simulink model "Calibration_IcestorageModel"  (R2018b)
settings: Solver=ode45  StartTime=(-31+16)*24*3600*0  StopTime=(31+29+31+30+31+30+31+31)*24*3600 %23*24*3600  EnableMultiTasking=on
libraries: carnot x43
(part 2 of 2)

== system Calibration_IcestorageModel/Daten Ldf einlesen messdaten1_2011dez_2012aug/InteressanterRest ==
  data : Inport
  Selector : Selector  InputPortWidth=36  IndexOptions=Index vector (dialog)  Indices=[v]  OutputSizes=1
  out : Outport  InitialOutput=0
  wires:
  data/1 -> Selector/1
  Selector/1 -> out/1

== system Calibration_IcestorageModel/Daten Ldf einlesen messdaten1_2011dez_2012aug/InteressanterRest1 ==
  data : Inport
  Selector : Selector  InputPortWidth=36  IndexOptions=Index vector (dialog)  Indices=[v]  OutputSizes=1
  out : Outport  InitialOutput=0
  wires:
  Selector/1 -> out/1
  data/1 -> Selector/1

== system Calibration_IcestorageModel/Daten Ldf einlesen messdaten1_2011dez_2012aug/InteressanterRest2 ==
  data : Inport
  Selector : Selector  InputPortWidth=36  IndexOptions=Index vector (dialog)  Indices=[v]  OutputSizes=1
  out : Outport  InitialOutput=0
  wires:
  data/1 -> Selector/1
  Selector/1 -> out/1

== system Calibration_IcestorageModel/Daten Ldf einlesen messdaten1_2011dez_2012aug/InteressanterRest3 ==
  data : Inport
  Selector : Selector  InputPortWidth=36  IndexOptions=Index vector (dialog)  Indices=[v]  OutputSizes=1
  out : Outport  InitialOutput=0
  wires:
  Selector/1 -> out/1
  data/1 -> Selector/1

== system Calibration_IcestorageModel/Daten Ldf einlesen messdaten1_2011dez_2012aug/Strom ==
  data : Inport
  Selector : Selector  InputPortWidth=36  IndexOptions=Index vector (dialog)  Indices=[v]  OutputSizes=1
  out : Outport  InitialOutput=0
  wires:
  Selector/1 -> out/1
  data/1 -> Selector/1

== system Calibration_IcestorageModel/Daten Ldf einlesen messdaten1_2011dez_2012aug/THO ==
  data : Inport
  Selector : Selector  InputPortWidth=36  IndexOptions=Index vector (dialog)  Indices=[v]  OutputSizes=1
  out : Outport  InitialOutput=0
  wires:
  Selector/1 -> out/1
  data/1 -> Selector/1

== system Calibration_IcestorageModel/Daten Ldf einlesen messdaten1_2011dez_2012aug/converts 4-20mA  to  0-1500W ==
  note: converts
      | 4-20mA  to  0-1500W
  In1 : Inport
  Bias : Bias  Bias=-0.0041
  Gain : Gain  Gain=1/0.0159*1500
  Out1 : Outport
  wires:
  Gain/1 -> Out1/1
  In1/1 -> Bias/1
  Bias/1 -> Gain/1

== system Calibration_IcestorageModel/ice_storage earth-mdl r05/heat exchanger heat pump ==
  Tice : Inport
  Tin : Inport  Port=2
  mdot : Inport  Port=3
  p : Inport  Port=4
  fluid : Inport  Port=5
  mix : Inport  Port=6
  1/(m*cp) : Gain  Gain=1/(1*l_hp*3500)  SaturateOnIntegerOverflow=on  OutDataTypeStr=Inherit: Same as input  ParamDataTypeStr=Inherit: Same as input
  Integrator : Integrator
  Product : Product  Inputs=3  SaturateOnIntegerOverflow=on  InputSameDT=on  OutDataTypeStr=Inherit: Same as first input
  Sum : Sum  Inputs=-+  SaturateOnIntegerOverflow=on  InputSameDT=on  OutDataTypeStr=Inherit: Same as first input
  Sum1 : Sum  Inputs=-+  SaturateOnIntegerOverflow=on  InputSameDT=on  OutDataTypeStr=Inherit: Same as first input
  Sum2 : Sum  Inputs=+-  SaturateOnIntegerOverflow=on  InputSameDT=on  OutDataTypeStr=Inherit: Same as first input
  UA : Gain  Gain="1500/28/9.5*l_hp*25/32            % 1.5 kW at 9 K on a 28 m tube with Da=32 (now Da=25)"  SaturateOnIntegerOverflow=on  OutDataTypeStr=Inherit: Same as input  ParamDataTypeStr=Inherit: Same as input
  heat_capacity : carnot/Basic/Material_Properties/Heat_Capacity  VariantControl=CarlibClassic  INPUTARGUMENTS=state variables (classic)  DEBUGLEVEL=DEBUGLEVEL  MAXTOTALWARNINGS=inf  MAXCONSECUTIVEWARNINGS=inf  WRITETOFILE=0  FILENAME='errors.txt'
      settings: SourceProductName=Carnot
  Qdot2ice : Outport
  Thx_coll : Outport  Port=2
  wires:
  Tin/1 -> Sum/2, heat_capacity/1
  Integrator/1 -> Sum/1, Sum2/1, Thx_coll/1  "Thx_coll"
  Sum1/1 -> 1/(m*cp)/1
  Product/1 -> Sum1/2
  heat_capacity/1 -> Product/3
  Sum/1 -> Product/1
  Sum2/1 -> UA/1
  mdot/1 -> Product/2
  p/1 -> heat_capacity/2
  fluid/1 -> heat_capacity/3
  mix/1 -> heat_capacity/4
  Tice/1 -> Sum2/2
  1/(m*cp)/1 -> Integrator/1
  UA/1 -> Sum1/1, Qdot2ice/1

== system Calibration_IcestorageModel/ice_storage earth-mdl r05/heat exchanger solar ==
  Tice : Inport
  Tin : Inport  Port=2
  mdot : Inport  Port=3
  p : Inport  Port=4
  fluid : Inport  Port=5
  mix : Inport  Port=6
  1/(m*cp) : Gain  Gain=1/(1*l_solar*3500)  SaturateOnIntegerOverflow=on  OutDataTypeStr=Inherit: Same as input  ParamDataTypeStr=Inherit: Same as input
  Integrator : Integrator
  Product : Product  Inputs=3  SaturateOnIntegerOverflow=on  InputSameDT=on  OutDataTypeStr=Inherit: Same as first input
  Sum : Sum  Inputs=-+  SaturateOnIntegerOverflow=on  InputSameDT=on  OutDataTypeStr=Inherit: Same as first input
  Sum1 : Sum  Inputs=-+  SaturateOnIntegerOverflow=on  InputSameDT=on  OutDataTypeStr=Inherit: Same as first input
  Sum2 : Sum  Inputs=+-  SaturateOnIntegerOverflow=on  InputSameDT=on  OutDataTypeStr=Inherit: Same as first input
  UA : Gain  Gain="1500/28/9.5*l_solar*25/32            % 1.5 kW at 9 K on a 28 m tube with Da=32 (now Da=25)"  SaturateOnIntegerOverflow=on  OutDataTypeStr=Inherit: Same as input  ParamDataTypeStr=Inherit: Same as input
  heat_capacity : carnot/Basic/Material_Properties/Heat_Capacity  VariantControl=CarlibClassic  INPUTARGUMENTS=state variables (classic)  DEBUGLEVEL=DEBUGLEVEL  MAXTOTALWARNINGS=inf  MAXCONSECUTIVEWARNINGS=inf  WRITETOFILE=0  FILENAME='errors.txt'
      settings: SourceProductName=Carnot
  Qdot2ice : Outport
  Thx_coll : Outport  Port=2
  wires:
  Tice/1 -> Sum2/2
  mix/1 -> heat_capacity/4
  fluid/1 -> heat_capacity/3
  p/1 -> heat_capacity/2
  mdot/1 -> Product/2
  Sum2/1 -> UA/1
  Sum/1 -> Product/1
  heat_capacity/1 -> Product/3
  Product/1 -> Sum1/2
  Sum1/1 -> 1/(m*cp)/1
  Integrator/1 -> Thx_coll/1, Sum2/1, Sum/1  "Thx_coll"
  Tin/1 -> heat_capacity/1, Sum/2
  1/(m*cp)/1 -> Integrator/1
  UA/1 -> Qdot2ice/1, Sum1/1

== system Calibration_IcestorageModel/ice_storage earth-mdl r05/undisturbed ground temperature1 ==
  Fcn : Fcn  Expr=u(1) - u(2)*exp(-u(3)/u(4))*cos(2*pi*(u(5)-u(6)*3600)/(365*24*3600) - u(3)/u(4)) + 0.03*u(3)
  Mux : Mux  Inputs=6
  Tmeanoutside : Constant  Value=Tmeanoutside
  delta_grd : Constant  Value=delta_grd
  deltathetae : Constant  Value=deltathetae
  depth of center of wall : Constant  Value=ztilde
  time : Clock
  tshift : Constant  Value=tshift
  Tearth : Outport
  wires:
  Fcn/1 -> Tearth/1
  Mux/1 -> Fcn/1
  tshift/1 -> Mux/6
  time/1 -> Mux/5
  delta_grd/1 -> Mux/4
  depth of center of wall/1 -> Mux/3
  deltathetae/1 -> Mux/2
  Tmeanoutside/1 -> Mux/1

== system Calibration_IcestorageModel/ice_storage new earth+HX-mdl_r06/heat exchanger solar ==
  Tice : Inport
  Tin : Inport  Port=2
  mdot : Inport  Port=3
  p : Inport  Port=4
  fluid : Inport  Port=5
  mix : Inport  Port=6
  1/(m*cp) : Gain  Gain=1/(1*l_solar*3500)  SaturateOnIntegerOverflow=on  OutDataTypeStr=Inherit: Same as input  ParamDataTypeStr=Inherit: Same as input
  Integrator : Integrator
  Product : Product  Inputs=3  SaturateOnIntegerOverflow=on  InputSameDT=on  OutDataTypeStr=Inherit: Same as first input
  Sum : Sum  Inputs=-+  SaturateOnIntegerOverflow=on  InputSameDT=on  OutDataTypeStr=Inherit: Same as first input
  Sum1 : Sum  Inputs=-+  SaturateOnIntegerOverflow=on  InputSameDT=on  OutDataTypeStr=Inherit: Same as first input
  Sum2 : Sum  Inputs=+-  SaturateOnIntegerOverflow=on  InputSameDT=on  OutDataTypeStr=Inherit: Same as first input
  UA : Gain  Gain="1500/28/9.5*l_solar*25/32            % 1.5 kW at 9 K on a 28 m tube with Da=32 (now Da=25)"  SaturateOnIntegerOverflow=on  OutDataTypeStr=Inherit: Same as input  ParamDataTypeStr=Inherit: Same as input
  heat_capacity : carnot/Basic/Material_Properties/Heat_Capacity  VariantControl=CarlibClassic  INPUTARGUMENTS=state variables (classic)  DEBUGLEVEL=DEBUGLEVEL  MAXTOTALWARNINGS=inf  MAXCONSECUTIVEWARNINGS=inf  WRITETOFILE=0  FILENAME='errors.txt'
      settings: SourceProductName=Carnot
  Qdot2ice : Outport
  Thx_coll : Outport  Port=2
  wires:
  Tin/1 -> Sum/2, heat_capacity/1
  Integrator/1 -> Sum/1, Sum2/1, Thx_coll/1  "Thx_coll"
  1/(m*cp)/1 -> Integrator/1
  Sum1/1 -> 1/(m*cp)/1
  Product/1 -> Sum1/2
  heat_capacity/1 -> Product/3
  Sum/1 -> Product/1
  Sum2/1 -> UA/1
  UA/1 -> Qdot2ice/1, Sum1/1
  mdot/1 -> Product/2
  p/1 -> heat_capacity/2
  fluid/1 -> heat_capacity/3
  mix/1 -> heat_capacity/4
  Tice/1 -> Sum2/2

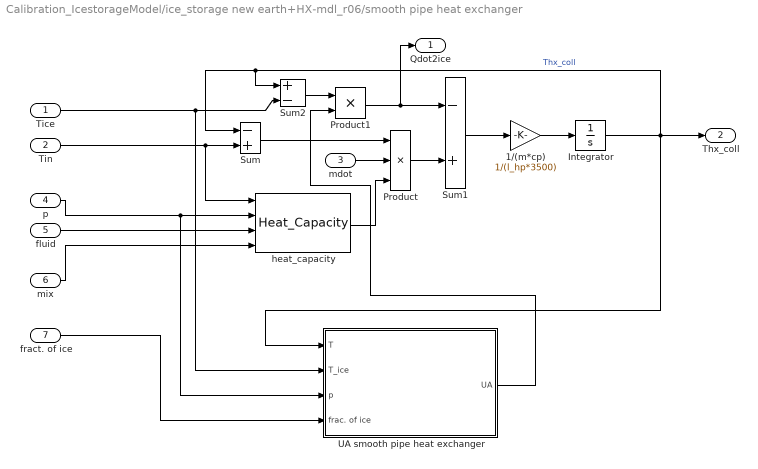
== system Calibration_IcestorageModel/ice_storage new earth+HX-mdl_r06/smooth pipe heat exchanger ==
  Tice : Inport
  Tin : Inport  Port=2
  mdot : Inport  Port=3
  p : Inport  Port=4
  fluid : Inport  Port=5
  mix : Inport  Port=6
  fract. of ice : Inport  Port=7
  1/(m*cp) : Gain  Gain=1/(l_hp*3500)  SaturateOnIntegerOverflow=on  OutDataTypeStr=Inherit: Same as input  ParamDataTypeStr=Inherit: Same as input
  Integrator : Integrator
  Product : Product  Inputs=3  SaturateOnIntegerOverflow=on  InputSameDT=on  OutDataTypeStr=Inherit: Same as first input
  Product1 : Product  RndMeth=Zero
  Sum : Sum  Inputs=-+  SaturateOnIntegerOverflow=on  InputSameDT=on  OutDataTypeStr=Inherit: Same as first input
  Sum1 : Sum  Inputs=-+  SaturateOnIntegerOverflow=on  InputSameDT=on  OutDataTypeStr=Inherit: Same as first input
  Sum2 : Sum  Inputs=+-  SaturateOnIntegerOverflow=on  InputSameDT=on  OutDataTypeStr=Inherit: Same as first input
  UA smooth pipe heat exchanger : Subsystem
      mask help:
      | Calculates the  heat exchange of a smooth pipe heat exchanger.
      | Calls calls the function "grashof" in the CARNOT library "carlib".
      | Definition of the fluid types
      | fluid-ID  material           remarks on fluid mix
      | 1           water              vapourcontent in the 2-phase region
      | 2           air                   is (kg water) / (kg air)
      | 3           cotton oil
      | 4           silicone oil
      | 5           water-glycol    gives the volume partition [0..1] of glycol
  heat_capacity : carnot/Basic/Material_Properties/Heat_Capacity  VariantControl=CarlibClassic  INPUTARGUMENTS=state variables (classic)  DEBUGLEVEL=DEBUGLEVEL  MAXTOTALWARNINGS=inf  MAXCONSECUTIVEWARNINGS=inf  WRITETOFILE=0  FILENAME='errors.txt'
      settings: SourceProductName=Carnot
  Qdot2ice : Outport
  Thx_coll : Outport  Port=2
  wires:
  fract. of ice/1 -> UA smooth pipe heat exchanger/4(frac. of ice)
  Product1/1 -> Sum1/1, Qdot2ice/1
  UA smooth pipe heat exchanger/1(UA) -> Product1/2
  Tin/1 -> Sum/2, heat_capacity/1
  Integrator/1 -> Sum/1, Sum2/1, Thx_coll/1, UA smooth pipe heat exchanger/1(T)  "Thx_coll"
  Sum1/1 -> 1/(m*cp)/1
  Product/1 -> Sum1/2
  heat_capacity/1 -> Product/3
  Sum/1 -> Product/1
  Sum2/1 -> Product1/1
  mdot/1 -> Product/2
  p/1 -> UA smooth pipe heat exchanger/3(p), heat_capacity/2
  fluid/1 -> heat_capacity/3
  mix/1 -> heat_capacity/4
  Tice/1 -> UA smooth pipe heat exchanger/2(T_ice), Sum2/2
  1/(m*cp)/1 -> Integrator/1

== system Calibration_IcestorageModel/ice_storage new earth+HX-mdl_r06/undisturbed ground temperature ==
  Fcn : Fcn  Expr=u(1) - u(2)*exp(-u(3)/u(4))*cos(2*pi*(u(5)-u(6)*3600)/(365*24*3600) - u(3)/u(4)) + 0.03*u(3)
  Mux : Mux  Inputs=6
  Tmeanoutside : Constant  Value=Tmeanoutside
  delta_grd : Constant  Value=delta_grd
  deltathetae : Constant  Value=deltathetae
  depth of center of wall : Constant  Value=ztilde
  time : Clock
  tshift : Constant  Value=tshift
  Tearth : Outport
  wires:
  Fcn/1 -> Tearth/1
  Mux/1 -> Fcn/1
  tshift/1 -> Mux/6
  time/1 -> Mux/5
  delta_grd/1 -> Mux/4
  depth of center of wall/1 -> Mux/3
  deltathetae/1 -> Mux/2
  Tmeanoutside/1 -> Mux/1

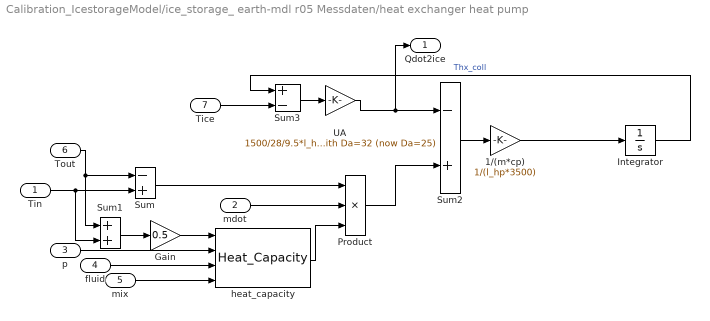
== system Calibration_IcestorageModel/ice_storage_ earth-mdl r05 Messdaten/heat exchanger heat pump ==
  Tin : Inport
  mdot : Inport  Port=2
  p : Inport  Port=3
  fluid : Inport  Port=4
  mix : Inport  Port=5
  Tout : Inport  Port=6
  Tice : Inport  Port=7
  1/(m*cp) : Gain  Gain=1/(l_hp*3500)  SaturateOnIntegerOverflow=on  OutDataTypeStr=Inherit: Same as input  ParamDataTypeStr=Inherit: Same as input
  Gain : Gain  Gain=0.5
  Integrator : Integrator
  Product : Product  Inputs=3  SaturateOnIntegerOverflow=on  InputSameDT=on  OutDataTypeStr=Inherit: Same as first input
  Sum : Sum  Inputs=-+  SaturateOnIntegerOverflow=on  InputSameDT=on  OutDataTypeStr=Inherit: Same as first input
  Sum1 : Sum  SaturateOnIntegerOverflow=on  InputSameDT=on  OutDataTypeStr=Inherit: Same as first input
  Sum2 : Sum  Inputs=-+  SaturateOnIntegerOverflow=on  InputSameDT=on  OutDataTypeStr=Inherit: Same as first input
  Sum3 : Sum  Inputs=+-  SaturateOnIntegerOverflow=on  InputSameDT=on  OutDataTypeStr=Inherit: Same as first input
  UA : Gain  Gain="1500/28/9.5*l_hp*25/32            % 1.5 kW at 9 K on a 28 m tube with Da=32 (now Da=25)"  SaturateOnIntegerOverflow=on  OutDataTypeStr=Inherit: Same as input  ParamDataTypeStr=Inherit: Same as input
  heat_capacity : carnot/Basic/Material_Properties/Heat_Capacity  VariantControl=CarlibClassic  INPUTARGUMENTS=state variables (classic)  DEBUGLEVEL=DEBUGLEVEL  MAXTOTALWARNINGS=inf  MAXCONSECUTIVEWARNINGS=inf  WRITETOFILE=0  FILENAME='errors.txt'
      settings: SourceProductName=Carnot
  Qdot2ice : Outport
  wires:
  Gain/1 -> heat_capacity/1
  Sum1/1 -> Gain/1
  Tout/1 -> Sum1/1, Sum/1
  Tin/1 -> Sum1/2, Sum/2
  heat_capacity/1 -> Product/3
  Sum/1 -> Product/1
  mdot/1 -> Product/2
  p/1 -> heat_capacity/2
  fluid/1 -> heat_capacity/3
  mix/1 -> heat_capacity/4
  UA/1 -> Sum2/1, Qdot2ice/1
  Integrator/1 -> Sum3/1  "Thx_coll"
  Sum2/1 -> 1/(m*cp)/1
  Sum3/1 -> UA/1
  1/(m*cp)/1 -> Integrator/1
  Product/1 -> Sum2/2
  Tice/1 -> Sum3/2

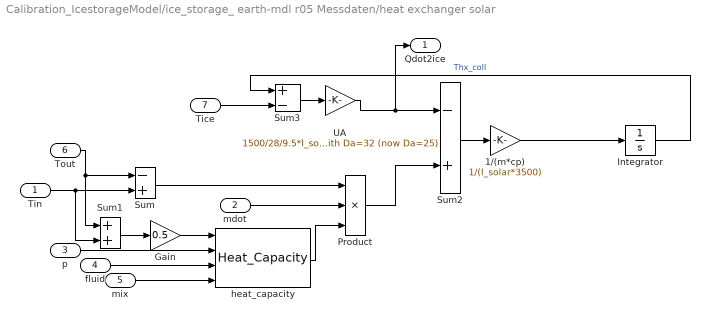
== system Calibration_IcestorageModel/ice_storage_ earth-mdl r05 Messdaten/heat exchanger solar ==
  Tin : Inport
  mdot : Inport  Port=2
  p : Inport  Port=3
  fluid : Inport  Port=4
  mix : Inport  Port=5
  Tout : Inport  Port=6
  Tice : Inport  Port=7
  1/(m*cp) : Gain  Gain=1/(l_solar*3500)  SaturateOnIntegerOverflow=on  OutDataTypeStr=Inherit: Same as input  ParamDataTypeStr=Inherit: Same as input
  Gain : Gain  Gain=0.5
  Integrator : Integrator
  Product : Product  Inputs=3  SaturateOnIntegerOverflow=on  InputSameDT=on  OutDataTypeStr=Inherit: Same as first input
  Sum : Sum  Inputs=-+  SaturateOnIntegerOverflow=on  InputSameDT=on  OutDataTypeStr=Inherit: Same as first input
  Sum1 : Sum  SaturateOnIntegerOverflow=on  InputSameDT=on  OutDataTypeStr=Inherit: Same as first input
  Sum2 : Sum  Inputs=-+  SaturateOnIntegerOverflow=on  InputSameDT=on  OutDataTypeStr=Inherit: Same as first input
  Sum3 : Sum  Inputs=+-  SaturateOnIntegerOverflow=on  InputSameDT=on  OutDataTypeStr=Inherit: Same as first input
  UA : Gain  Gain="1500/28/9.5*l_solar*25/32            % 1.5 kW at 9 K on a 28 m tube with Da=32 (now Da=25)"  SaturateOnIntegerOverflow=on  OutDataTypeStr=Inherit: Same as input  ParamDataTypeStr=Inherit: Same as input
  heat_capacity : carnot/Basic/Material_Properties/Heat_Capacity  VariantControl=CarlibClassic  INPUTARGUMENTS=state variables (classic)  DEBUGLEVEL=DEBUGLEVEL  MAXTOTALWARNINGS=inf  MAXCONSECUTIVEWARNINGS=inf  WRITETOFILE=0  FILENAME='errors.txt'
      settings: SourceProductName=Carnot
  Qdot2ice : Outport
  wires:
  Tice/1 -> Sum3/2
  Product/1 -> Sum2/2
  1/(m*cp)/1 -> Integrator/1
  Sum3/1 -> UA/1
  Sum2/1 -> 1/(m*cp)/1
  Integrator/1 -> Sum3/1  "Thx_coll"
  UA/1 -> Qdot2ice/1, Sum2/1
  mix/1 -> heat_capacity/4
  fluid/1 -> heat_capacity/3
  p/1 -> heat_capacity/2
  mdot/1 -> Product/2
  Sum/1 -> Product/1
  heat_capacity/1 -> Product/3
  Tin/1 -> Sum/2, Sum1/2
  Tout/1 -> Sum/1, Sum1/1
  Sum1/1 -> Gain/1
  Gain/1 -> heat_capacity/1

== system Calibration_IcestorageModel/ice_storage_ earth-mdl r05 Messdaten/undisturbed ground temperature1 ==
  Fcn : Fcn  Expr=u(1) - u(2)*exp(-u(3)/u(4))*cos(2*pi*(u(5)-u(6)*3600)/(365*24*3600) - u(3)/u(4)) + 0.03*u(3)
  Mux : Mux  Inputs=6
  Tmeanoutside : Constant  Value=Tmeanoutside
  delta_grd : Constant  Value=delta_grd
  deltathetae : Constant  Value=deltathetae
  depth of center of wall : Constant  Value=ztilde
  time : Clock
  tshift : Constant  Value=tshift
  Tearth : Outport
  wires:
  Fcn/1 -> Tearth/1
  Mux/1 -> Fcn/1
  tshift/1 -> Mux/6
  time/1 -> Mux/5
  delta_grd/1 -> Mux/4
  depth of center of wall/1 -> Mux/3
  deltathetae/1 -> Mux/2
  Tmeanoutside/1 -> Mux/1

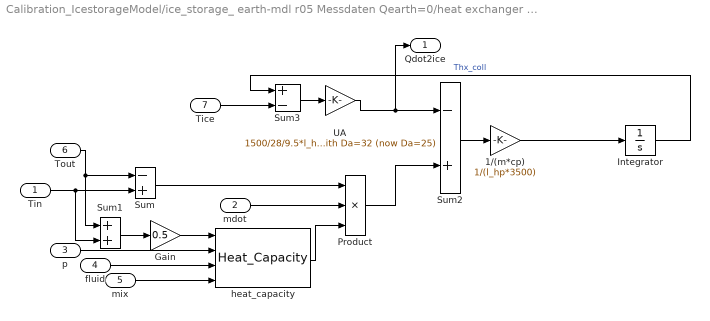
== system Calibration_IcestorageModel/ice_storage_ earth-mdl r05 Messdaten Qearth=0/heat exchanger heat pump ==
  Tin : Inport
  mdot : Inport  Port=2
  p : Inport  Port=3
  fluid : Inport  Port=4
  mix : Inport  Port=5
  Tout : Inport  Port=6
  Tice : Inport  Port=7
  1/(m*cp) : Gain  Gain=1/(l_hp*3500)  SaturateOnIntegerOverflow=on  OutDataTypeStr=Inherit: Same as input  ParamDataTypeStr=Inherit: Same as input
  Gain : Gain  Gain=0.5
  Integrator : Integrator
  Product : Product  Inputs=3  SaturateOnIntegerOverflow=on  InputSameDT=on  OutDataTypeStr=Inherit: Same as first input
  Sum : Sum  Inputs=-+  SaturateOnIntegerOverflow=on  InputSameDT=on  OutDataTypeStr=Inherit: Same as first input
  Sum1 : Sum  SaturateOnIntegerOverflow=on  InputSameDT=on  OutDataTypeStr=Inherit: Same as first input
  Sum2 : Sum  Inputs=-+  SaturateOnIntegerOverflow=on  InputSameDT=on  OutDataTypeStr=Inherit: Same as first input
  Sum3 : Sum  Inputs=+-  SaturateOnIntegerOverflow=on  InputSameDT=on  OutDataTypeStr=Inherit: Same as first input
  UA : Gain  Gain="1500/28/9.5*l_hp*25/32            % 1.5 kW at 9 K on a 28 m tube with Da=32 (now Da=25)"  SaturateOnIntegerOverflow=on  OutDataTypeStr=Inherit: Same as input  ParamDataTypeStr=Inherit: Same as input
  heat_capacity : carnot/Basic/Material_Properties/Heat_Capacity  VariantControl=CarlibClassic  INPUTARGUMENTS=state variables (classic)  DEBUGLEVEL=DEBUGLEVEL  MAXTOTALWARNINGS=inf  MAXCONSECUTIVEWARNINGS=inf  WRITETOFILE=0  FILENAME='errors.txt'
      settings: SourceProductName=Carnot
  Qdot2ice : Outport
  wires:
  Tice/1 -> Sum3/2
  Product/1 -> Sum2/2
  1/(m*cp)/1 -> Integrator/1
  Sum3/1 -> UA/1
  Sum2/1 -> 1/(m*cp)/1
  Integrator/1 -> Sum3/1  "Thx_coll"
  UA/1 -> Qdot2ice/1, Sum2/1
  mix/1 -> heat_capacity/4
  fluid/1 -> heat_capacity/3
  p/1 -> heat_capacity/2
  mdot/1 -> Product/2
  Sum/1 -> Product/1
  heat_capacity/1 -> Product/3
  Tin/1 -> Sum/2, Sum1/2
  Tout/1 -> Sum/1, Sum1/1
  Sum1/1 -> Gain/1
  Gain/1 -> heat_capacity/1

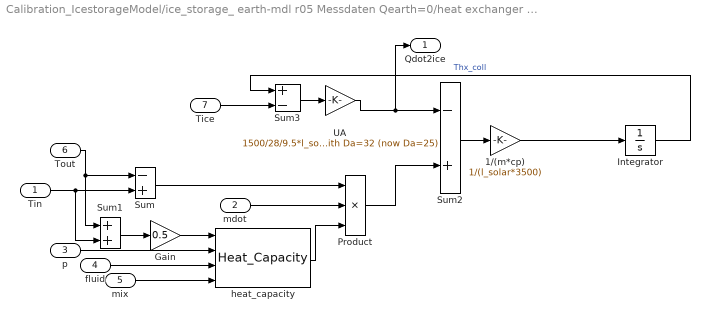
== system Calibration_IcestorageModel/ice_storage_ earth-mdl r05 Messdaten Qearth=0/heat exchanger solar ==
  Tin : Inport
  mdot : Inport  Port=2
  p : Inport  Port=3
  fluid : Inport  Port=4
  mix : Inport  Port=5
  Tout : Inport  Port=6
  Tice : Inport  Port=7
  1/(m*cp) : Gain  Gain=1/(l_solar*3500)  SaturateOnIntegerOverflow=on  OutDataTypeStr=Inherit: Same as input  ParamDataTypeStr=Inherit: Same as input
  Gain : Gain  Gain=0.5
  Integrator : Integrator
  Product : Product  Inputs=3  SaturateOnIntegerOverflow=on  InputSameDT=on  OutDataTypeStr=Inherit: Same as first input
  Sum : Sum  Inputs=-+  SaturateOnIntegerOverflow=on  InputSameDT=on  OutDataTypeStr=Inherit: Same as first input
  Sum1 : Sum  SaturateOnIntegerOverflow=on  InputSameDT=on  OutDataTypeStr=Inherit: Same as first input
  Sum2 : Sum  Inputs=-+  SaturateOnIntegerOverflow=on  InputSameDT=on  OutDataTypeStr=Inherit: Same as first input
  Sum3 : Sum  Inputs=+-  SaturateOnIntegerOverflow=on  InputSameDT=on  OutDataTypeStr=Inherit: Same as first input
  UA : Gain  Gain="1500/28/9.5*l_solar*25/32            % 1.5 kW at 9 K on a 28 m tube with Da=32 (now Da=25)"  SaturateOnIntegerOverflow=on  OutDataTypeStr=Inherit: Same as input  ParamDataTypeStr=Inherit: Same as input
  heat_capacity : carnot/Basic/Material_Properties/Heat_Capacity  VariantControl=CarlibClassic  INPUTARGUMENTS=state variables (classic)  DEBUGLEVEL=DEBUGLEVEL  MAXTOTALWARNINGS=inf  MAXCONSECUTIVEWARNINGS=inf  WRITETOFILE=0  FILENAME='errors.txt'
      settings: SourceProductName=Carnot
  Qdot2ice : Outport
  wires:
  Gain/1 -> heat_capacity/1
  Sum1/1 -> Gain/1
  Tout/1 -> Sum1/1, Sum/1
  Tin/1 -> Sum1/2, Sum/2
  heat_capacity/1 -> Product/3
  Sum/1 -> Product/1
  mdot/1 -> Product/2
  p/1 -> heat_capacity/2
  fluid/1 -> heat_capacity/3
  mix/1 -> heat_capacity/4
  UA/1 -> Sum2/1, Qdot2ice/1
  Integrator/1 -> Sum3/1  "Thx_coll"
  Sum2/1 -> 1/(m*cp)/1
  Sum3/1 -> UA/1
  1/(m*cp)/1 -> Integrator/1
  Product/1 -> Sum2/2
  Tice/1 -> Sum3/2

== system Calibration_IcestorageModel/ice_storage_ earth-mdl r05 Messdaten Qearth=0/undisturbed ground temperature1 ==
  Fcn : Fcn  Expr=u(1) - u(2)*exp(-u(3)/u(4))*cos(2*pi*(u(5)-u(6)*3600)/(365*24*3600) - u(3)/u(4)) + 0.03*u(3)
  Mux : Mux  Inputs=6
  Tmeanoutside : Constant  Value=Tmeanoutside
  delta_grd : Constant  Value=delta_grd
  deltathetae : Constant  Value=deltathetae
  depth of center of wall : Constant  Value=ztilde
  time : Clock
  tshift : Constant  Value=tshift
  Tearth : Outport
  wires:
  Tmeanoutside/1 -> Mux/1
  deltathetae/1 -> Mux/2
  depth of center of wall/1 -> Mux/3
  delta_grd/1 -> Mux/4
  time/1 -> Mux/5
  tshift/1 -> Mux/6
  Mux/1 -> Fcn/1
  Fcn/1 -> Tearth/1

== system Calibration_IcestorageModel/ice_storage_r04 Messdaten/heat exchanger heat pump ==
  Tin : Inport
  mdot : Inport  Port=2
  p : Inport  Port=3
  fluid : Inport  Port=4
  mix : Inport  Port=5
  Tout : Inport  Port=6
  Tice : Inport  Port=7
  1/(m*cp) : Gain  Gain=1/(l_hp*3500)  SaturateOnIntegerOverflow=on  OutDataTypeStr=Inherit: Same as input  ParamDataTypeStr=Inherit: Same as input
  Gain : Gain  Gain=0.5
  Integrator : Integrator
  Product : Product  Inputs=3  SaturateOnIntegerOverflow=on  InputSameDT=on  OutDataTypeStr=Inherit: Same as first input
  Sum : Sum  Inputs=-+  SaturateOnIntegerOverflow=on  InputSameDT=on  OutDataTypeStr=Inherit: Same as first input
  Sum1 : Sum  SaturateOnIntegerOverflow=on  InputSameDT=on  OutDataTypeStr=Inherit: Same as first input
  Sum2 : Sum  Inputs=-+  SaturateOnIntegerOverflow=on  InputSameDT=on  OutDataTypeStr=Inherit: Same as first input
  Sum3 : Sum  Inputs=+-  SaturateOnIntegerOverflow=on  InputSameDT=on  OutDataTypeStr=Inherit: Same as first input
  UA : Gain  Gain="1500/28/9.5*l_hp*25/32            % 1.5 kW at 9 K on a 28 m tube with Da=32 (now Da=25)"  SaturateOnIntegerOverflow=on  OutDataTypeStr=Inherit: Same as input  ParamDataTypeStr=Inherit: Same as input
  heat_capacity : carnot/Basic/Material_Properties/Heat_Capacity  VariantControl=CarlibClassic  INPUTARGUMENTS=state variables (classic)  DEBUGLEVEL=DEBUGLEVEL  MAXTOTALWARNINGS=inf  MAXCONSECUTIVEWARNINGS=inf  WRITETOFILE=0  FILENAME='errors.txt'
      settings: SourceProductName=Carnot
  Qdot2ice : Outport
  wires:
  Gain/1 -> heat_capacity/1
  Sum1/1 -> Gain/1
  Tout/1 -> Sum1/1, Sum/1
  Tin/1 -> Sum1/2, Sum/2
  heat_capacity/1 -> Product/3
  Sum/1 -> Product/1
  mdot/1 -> Product/2
  p/1 -> heat_capacity/2
  fluid/1 -> heat_capacity/3
  mix/1 -> heat_capacity/4
  UA/1 -> Sum2/1, Qdot2ice/1
  Integrator/1 -> Sum3/1  "Thx_coll"
  Sum2/1 -> 1/(m*cp)/1
  Sum3/1 -> UA/1
  1/(m*cp)/1 -> Integrator/1
  Product/1 -> Sum2/2
  Tice/1 -> Sum3/2

== system Calibration_IcestorageModel/ice_storage_r04 Messdaten/heat exchanger solar ==
  Tin : Inport
  mdot : Inport  Port=2
  p : Inport  Port=3
  fluid : Inport  Port=4
  mix : Inport  Port=5
  Tout : Inport  Port=6
  Tice : Inport  Port=7
  1/(m*cp) : Gain  Gain=1/(l_solar*3500)  SaturateOnIntegerOverflow=on  OutDataTypeStr=Inherit: Same as input  ParamDataTypeStr=Inherit: Same as input
  Gain : Gain  Gain=0.5
  Integrator : Integrator
  Product : Product  Inputs=3  SaturateOnIntegerOverflow=on  InputSameDT=on  OutDataTypeStr=Inherit: Same as first input
  Sum : Sum  Inputs=-+  SaturateOnIntegerOverflow=on  InputSameDT=on  OutDataTypeStr=Inherit: Same as first input
  Sum1 : Sum  SaturateOnIntegerOverflow=on  InputSameDT=on  OutDataTypeStr=Inherit: Same as first input
  Sum2 : Sum  Inputs=-+  SaturateOnIntegerOverflow=on  InputSameDT=on  OutDataTypeStr=Inherit: Same as first input
  Sum3 : Sum  Inputs=+-  SaturateOnIntegerOverflow=on  InputSameDT=on  OutDataTypeStr=Inherit: Same as first input
  UA : Gain  Gain="1500/28/9.5*l_solar*25/32            % 1.5 kW at 9 K on a 28 m tube with Da=32 (now Da=25)"  SaturateOnIntegerOverflow=on  OutDataTypeStr=Inherit: Same as input  ParamDataTypeStr=Inherit: Same as input
  heat_capacity : carnot/Basic/Material_Properties/Heat_Capacity  VariantControl=CarlibClassic  INPUTARGUMENTS=state variables (classic)  DEBUGLEVEL=DEBUGLEVEL  MAXTOTALWARNINGS=inf  MAXCONSECUTIVEWARNINGS=inf  WRITETOFILE=0  FILENAME='errors.txt'
      settings: SourceProductName=Carnot
  Qdot2ice : Outport
  wires:
  Tice/1 -> Sum3/2
  Product/1 -> Sum2/2
  1/(m*cp)/1 -> Integrator/1
  Sum3/1 -> UA/1
  Sum2/1 -> 1/(m*cp)/1
  Integrator/1 -> Sum3/1  "Thx_coll"
  UA/1 -> Qdot2ice/1, Sum2/1
  mix/1 -> heat_capacity/4
  fluid/1 -> heat_capacity/3
  p/1 -> heat_capacity/2
  mdot/1 -> Product/2
  Sum/1 -> Product/1
  heat_capacity/1 -> Product/3
  Tin/1 -> Sum/2, Sum1/2
  Tout/1 -> Sum/1, Sum1/1
  Sum1/1 -> Gain/1
  Gain/1 -> heat_capacity/1

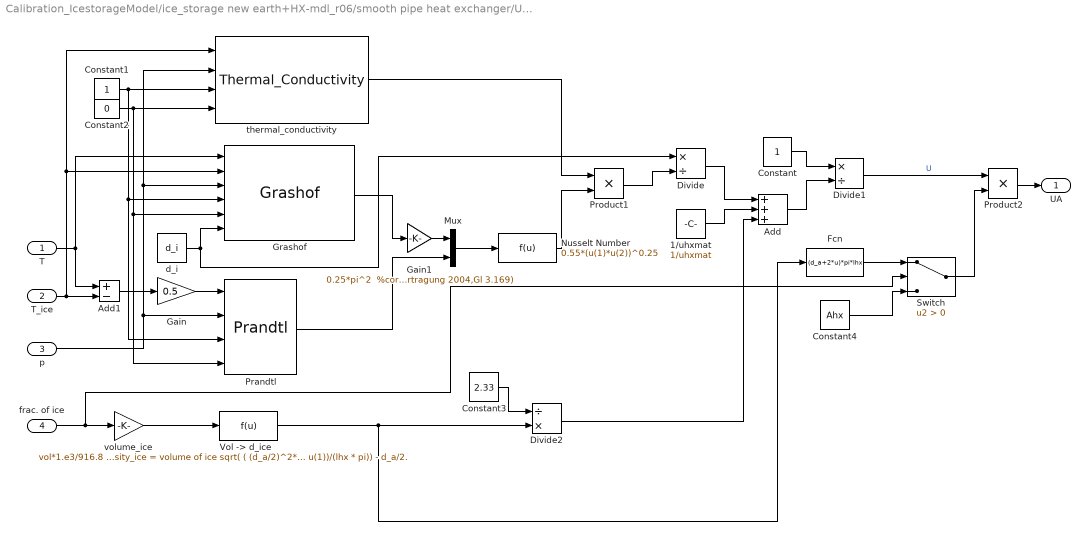
== system Calibration_IcestorageModel/ice_storage new earth+HX-mdl_r06/smooth pipe heat exchanger/UA smooth pipe heat exchanger ==
  T : Inport
  T_ice : Inport  Port=2
  p : Inport  Port=3
  frac. of ice : Inport  Port=4
  1/uhxmat : Constant  Value=1/uhxmat
  Add : Sum  Inputs=+++
  Add1 : Sum  Inputs=+-
  Constant : Constant
  Constant1 : Constant
  Constant2 : Constant  Value=0
  Constant3 : Constant  Value=2.33
  Constant4 : Constant  Value=Ahx
  Divide : Product  Inputs=*/
  Divide1 : Product  Inputs=*/
  Divide2 : Product  Inputs=/*
  Fcn : Fcn  Expr=(d_a+2*u)*pi*lhx
  Gain : Gain  Gain=0.5
  Gain1 : Gain  Gain="0.25*pi^2  %correction for horizontal pipe (Wagner Wärmeübertragung 2004,Gl 3.169)"
  Grashof : carnot/Basic/Hydraulics/Grashof  VariantControl=CarlibClassic  DEBUGLEVEL=WARNINGLEVEL  MAXTOTALMESSAGES=inf  MAXCONSECUTIVEMESSAGES=inf  WRITETOFILE=0  FILENAME='errors.txt'
      settings: SourceProductName=Carnot
  Mux : Mux  Inputs=2
  Nusselt Number : Fcn  Expr=0.55*(u(1)*u(2))^0.25
  Prandtl : carnot/Basic/Hydraulics/Prandtl  VariantControl=CarlibClassic  INPUTARGUMENTS=state variables (classic)  DEBUGLEVEL=WARNINGLEVEL  MAXTOTALMESSAGES=inf  MAXCONSECUTIVEMESSAGES=inf  WRITETOFILE=0  FILENAME='errors.txt'
      settings: SourceProductName=Carnot
  Product1 : Product  RndMeth=Zero
  Product2 : Product  RndMeth=Zero
  Switch : Switch  Criteria=u2 > Threshold
  "Vol -> d_ice" : Fcn  Expr=sqrt( ( (d_a/2)^2*pi*lhx + u(1))/(lhx * pi)) - d_a/2.
  d_i : Constant  Value=d_i
  thermal_conductivity : carnot/Basic/Material_Properties/Thermal_Conductivity  VariantControl=CarlibClassic  INPUTARGUMENTS=state variables (classic)  DEBUGLEVEL=WARNINGLEVEL  MAXTOTALMESSAGES=inf  MAXCONSECUTIVEMESSAGES=inf  WRITETOFILE=0  FILENAME='errors.txt'
      settings: SourceProductName=Carnot
  volume_ice : Gain  Gain=vol*1.e3/916.8 %volume*density_water/density_ice = volume of ice
  UA : Outport
  wires:
  Gain/1 -> Prandtl/1
  Gain1/1 -> Mux/1
  Divide2/1 -> Add/3
  "Vol -> d_ice"/1 -> Divide2/2, Fcn/1
  volume_ice/1 -> "Vol -> d_ice"/1
  frac. of ice/1 -> volume_ice/1, Switch/2
  Add1/1 -> Gain/1
  T/1 -> Grashof/1, Add1/1
  T_ice/1 -> Add1/2, Grashof/2, thermal_conductivity/1
  p/1 -> Prandtl/2, Grashof/3, thermal_conductivity/2
  d_i/1 -> Grashof/6, Divide/1
  Grashof/1 -> Gain1/1
  Prandtl/1 -> Mux/2
  Mux/1 -> Nusselt Number/1
  Nusselt Number/1 -> Product1/2
  Product1/1 -> Divide/2
  Divide/1 -> Add/1
  1/uhxmat/1 -> Add/2
  Constant/1 -> Divide1/1
  Add/1 -> Divide1/2
  Divide1/1 -> Product2/1  "U"
  Constant3/1 -> Divide2/1
  thermal_conductivity/1 -> Product1/1
  Constant1/1 -> thermal_conductivity/3, Prandtl/3, Grashof/4
  Constant2/1 -> thermal_conductivity/4, Prandtl/4, Grashof/5
  Product2/1 -> UA/1
  Fcn/1 -> Switch/1
  Constant4/1 -> Switch/3
  Switch/1 -> Product2/2
